simulink model "mass_spring_damp"  (R2020b)
settings: Solver=VariableStepAuto  StartTime=0.0  StopTime=10.0  RelTol=1e-3
values from neighbouring files (symbols this model uses):
  b = 50    [variable_declaration.m]
  k1 = 50    [variable_declaration.m]
  k12 = 25    [variable_declaration.m]
  m1 = 100    [variable_declaration.m]
  m2 = 50    [variable_declaration.m]
undefined symbols (not defined in the file or in its folder): k2
settings Model: Creator=shraddha  LastModifiedBy=shraddha

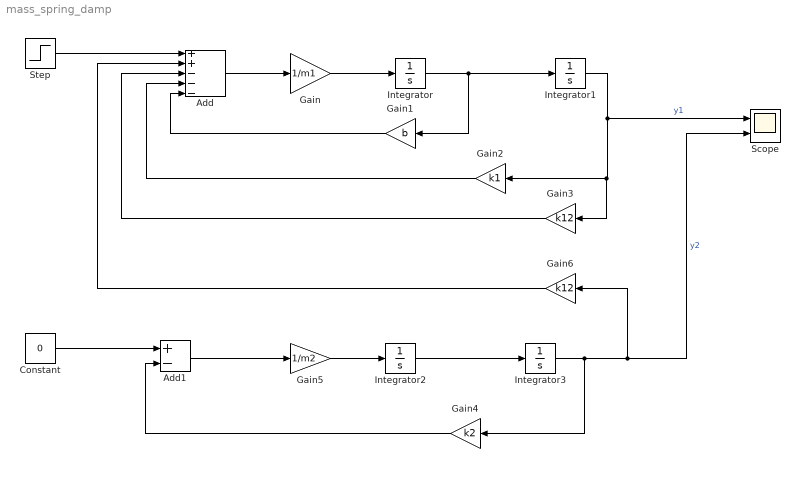
== system mass_spring_damp ==
  Add : Sum  Inputs=++---
  Add1 : Sum  Inputs=+-
  Constant : Constant  Value=0
  Gain : Gain  Gain=1/m1
  Gain1 : Gain  Gain=b
  Gain2 : Gain  Gain=k1
  Gain3 : Gain  Gain=k12
  Gain4 : Gain  Gain=k2
  Gain5 : Gain  Gain=1/m2
  Gain6 : Gain  Gain=k12
  Integrator{,1..3} (4 alike) : Integrator
  Scope : Scope  NumInputPorts=2
  Step : Step  SampleTime=0
  wires:
  Gain/1 -> Integrator/1
  Integrator/1 -> Gain1/1, Integrator1/1
  Integrator1/1 -> Gain3/1, Gain2/1, Scope/1  "y1"
  Gain5/1 -> Integrator2/1
  Integrator2/1 -> Integrator3/1
  Integrator3/1 -> Gain4/1, Gain6/1, Scope/2  "y2"
  Add/1 -> Gain/1
  Gain6/1 -> Add/2
  Gain1/1 -> Add/5
  Gain2/1 -> Add/4
  Gain3/1 -> Add/3
  Step/1 -> Add/1
  Add1/1 -> Gain5/1
  Gain4/1 -> Add1/2
  Constant/1 -> Add1/1
